simulink model "Vertiport_performance"  (R2022b)
settings: Solver=VariableStepAuto  StartTime=0.0  StopTime=1080  RelTol=1e-3
model workspace (MAT data in the model file):
  ChargingRate = 5
  MinTurnAround = 5
  ReqBatteryLevel = 70
  SeparationMinima = 3
  UAMDemand = 183
undefined symbols (not defined in the file or in its folder): entity, m, n, recordWaitTimes
settings Model: Creator=user  LastModifiedBy=user
settings SolverCC: AlgebraicLoopSolver=TrustRegion
settings DataIOCC: SaveOutput=off  SaveTime=off
settings DebuggingCC: UnconnectedInputMsg=warning  UnconnectedOutputMsg=warning  UnconnectedLineMsg=warning  SFMachineParentedDataDiag=warning  ArithmeticOperatorsInVariantConditions=warning
settings ModelReferenceCC: EnableRefExpFcnMdlSchedulingChecks=on
settings SFSimCC: SimUseLocalCustomCode=off  CustomCodeUndefinedFunction=UseInterfaceOnly
settings RTWCC: RTWUseLocalCustomCode=off
settings CodeAppCC: StateflowObjectComments=on

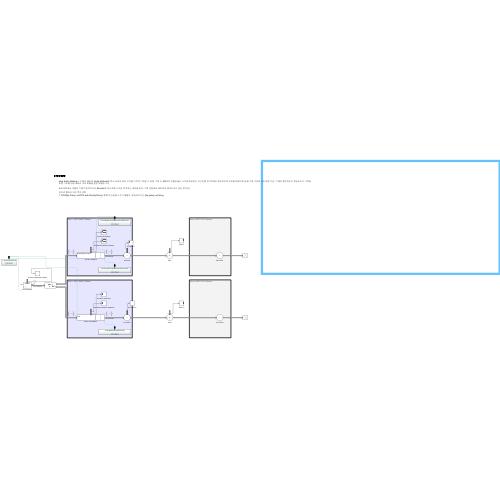
[thumbnail: Simulink's stored preview of the top-level diagram]
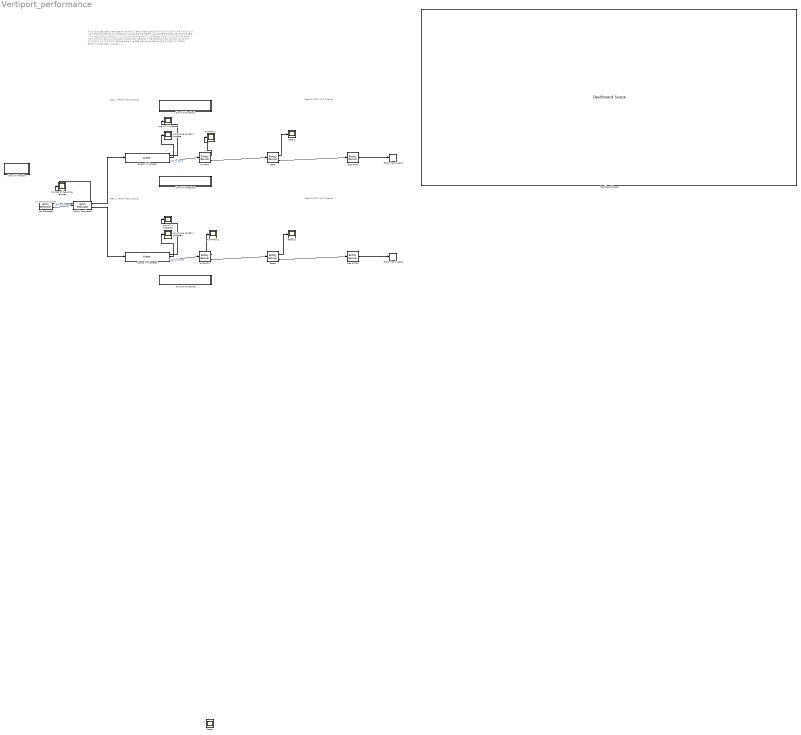
== system Vertiport_performance ==
  note: 27.7920676732485
  note: Step 3: FATO [·/D/1 Queue]
  note: Step 1: FATO [M/D/1 Queue]
  note: ※ 향후 방향
      |
      | Idea: Entity Attribute = 기체의 배터리, Entity Attribute에 따라 서버의 점유 시간을 다르게 가져갈 수 있음, 가령 1~100까지 만들어놓고 그거에 해당하는 시간만큼 게이트에서 점유하도록 규칙을 배정하면 실제 기체 거리에 따라 배정 가능. 기체의 충전속도는 동일하다고 가정 & 비행 거리에 따른 배터리 소모 비율을 알면 모델링 가능
      |
      | 버티포트에서 어떻게 기체가 움직이는지 Simulink로 모사해주고 이걸 분석하는 내용을 담자. 기체 관점에서 버티포트 에어사이드 성능 분석(?)
      |
      | 앞으로 뽑아야 하는 분석 방향
      | 1. FIFO(No Policy) vs FIFO with Priority(Policy): 통행 우선권을 가진 기체들의 평균대기시간 (No policy vs Policy),
  note: Step 1: FATO [M/D/1 Queue]
  note: Step 3: FATO [·/D/1 Queue]
  " Avg Queue Length in Airspace" : Scope
  " Avg Queue Length in Airspace1" : Scope
  Arr FATO : EntityServer  InputPortMessageModes=m  OutputPortMessageModes=n,m  Capacity=1  ServiceTimeSource=MATLAB action  ServiceTimeValue=1.5  ServiceTimeAction=dt = SeparationMinima;  Utilization=on
      settings: OutputPortMap=o5,o9
  Arr FATO U : Scope
  Arr FATO U1 : Scope
  Arr FATO1 : EntityServer  InputPortMessageModes=m  OutputPortMessageModes=n,m  Capacity=1  ServiceTimeSource=MATLAB action  ServiceTimeValue=1.5  ServiceTimeAction=dt = SeparationMinima;  Utilization=on
      settings: OutputPortMap=o5,o9
  Avg WT in Airspace : Scope
  Avg WT in Airspace1 : Scope
  Dashboard Scope : DashboardScope
  Dep FATO : EntityServer  InputPortMessageModes=m  OutputPortMessageModes=m  Capacity=1  ServiceTimeSource=MATLAB action  ServiceTimeAction=dt = SeparationMinima;
  Dep FATO1 : EntityServer  InputPortMessageModes=m  OutputPortMessageModes=m  Capacity=1  ServiceTimeSource=MATLAB action  ServiceTimeAction=dt = SeparationMinima;
  Entity Replicator : EntityReplicator  InputPortMessageModes=m  OutputPortMessageModes=m,m
  Entity Terminator1 : EntityTerminator  InputPortMessageModes=m
  Entity Terminator2 : EntityTerminator  InputPortMessageModes=m
  Gate : EntityServer  InputPortMessageModes=m  OutputPortMessageModes=n,m  ServiceTimeSource=MATLAB action  ServiceTimeValue=20  ServiceTimeAction=|  ServiceCompleteAction=|  Utilization=on
      ServiceTimeAction=|
      | if ReqBatteryLevel <= entity.Battery ...
      |         + MinTurnAround*ChargingRate
      |     dt = MinTurnAround;
      | else
      |     dt = (ReqBatteryLevel - entity.Battery)/ChargingRate
      | end
      ServiceCompleteAction=|
      | if entity.Battery >= ReqBatteryLevel - MinTurnAround*ChargingRate
      |     entity.Battery = min(100, entity.Battery + MinTurnAround*ChargingRate);
      | else
      |     entity.Battery = ReqBatteryLevel;
      | end
      settings: OutputPortMap=o5,o9
  Gate U : Scope
  Gate U1 : Scope
  Gate1 : EntityServer  InputPortMessageModes=m  OutputPortMessageModes=n,m  ServiceTimeSource=MATLAB action  ServiceTimeValue=20  ServiceTimeAction=|  ServiceCompleteAction=|  Utilization=on
      ServiceTimeAction=|
      | if ReqBatteryLevel <= entity.Battery ...
      |         + MinTurnAround*ChargingRate
      |     dt = MinTurnAround;
      | else
      |     dt = (ReqBatteryLevel - entity.Battery)/ChargingRate
      | end
      ServiceCompleteAction=|
      | if entity.Battery >= ReqBatteryLevel - MinTurnAround*ChargingRate
      |     entity.Battery = min(100, entity.Battery + MinTurnAround*ChargingRate);
      | else
      |     entity.Battery = ReqBatteryLevel;
      | end
      settings: OutputPortMap=o5,o9
  Number of departing vehicles : Scope
  Queue in Airspace : Queue  InputPortMessageModes=m  OutputPortMessageModes=n,n,m  Capacity=50  QueueType=Priority  PrioritySource=entitySys.priority  EntryAction=entity.StartTime = getCurrentTime();  ExitAction=|  AverageWait=on  AverageQueueLength=on
      | if entity.Class == 1
      |     recordHighPriorityWaitTimes(...
      |     entity.StartTime);
      | else
      |     recordLowPriorityWaitTimes(...
      |     entity.StartTime)
      | end % if entity.Class = 1
      settings: OutputPortMap=o2,o3,o5
  Queue in Airspace1 : Queue  InputPortMessageModes=m  OutputPortMessageModes=n,n,m  Capacity=50  PrioritySource=entitySys.priority  EntryAction=entity.StartTime = getCurrentTime();  ExitAction=recordWaitTimes(entity.StartTime)  AverageWait=on  AverageQueueLength=on
      settings: OutputPortMap=o2,o3,o5
  Simulink Function : Subsystem  TreatAsAtomicUnit=on
  Simulink Function1 : Subsystem  TreatAsAtomicUnit=on
  Simulink Function2 : Subsystem  TreatAsAtomicUnit=on
  Simulink Function5 : Subsystem  TreatAsAtomicUnit=on
  Veh Generator : EntityGenerator  OutputPortMessageModes=n,m  TimeSource=MATLAB action  IntergenerationTimeAction=|  GenerateEntityAtSimulationStart=off  GenerateAction=|  AttributeName=Battery|Class|StartTime  AttributeInitialValue=1|2|1  NumberEntitiesDeparted=on  EntityType=Structured  EntityTypeName=Vehicle
      IntergenerationTimeAction=|
      | persistent rngInit;
      | if isempty(rngInit)
      |     seed = 12345;
      |     rng(seed);
      |     rngInit = true;
      | end
      | 
      | B = [0.0361866444691084, 0.105565575286718, 0.157539076951535, 0.0409961154273030, 0.0182898631150573,0.0195847206807251, 0.0247930540140585, 0.0321113115057344, 0.0338628375878653, 0.0467131428042915, 0.0718472530521643, 0.0986172770995191, 0.121190575286718, 0.0568118756936737, 0.0477363115057344, 0.0432447743248243, 0.0326373473917869, 0.0122722438031817]';
      | Length = size(B,1);
      | UAMDemandHr = UAMDemand.*B(:,1);
      | Time = 60
      | Now = getCurrentTime();
      | aa = mod(Now, (Time*Length));
      | k = 1 + floor(aa./Time);
      | ArrivalRate = UAMDemandHr(k,1);
      | 
      | % Pattern: Exponential distribution
      | mu = 60/ArrivalRate; % mu = avg(interarrival time)
      | dt = - mu * log(1 - rand());
      GenerateAction=|
      | entity.Battery = randi(80);
      | % 배터리 1~80 까지 임의 생성
      | % 배터리 10미만이면 통행 우선권 부여
      | % 우버에서 minimum reserve 30%로 제
      | 
      | if entity.Battery <= 10
      |     entity.Class = 1;
      | else
      |     entity.Class = 2;
      | end % if entity.Battery < 10
      | 
      | entitySys.priority = entity.Class;
      settings: OutputPortMap=o0,o3
  Scope : Scope
  wires:
  Gate/2 -> Dep FATO/1
  Queue in Airspace/1 -> Avg WT in Airspace/1
  Arr FATO/2 -> Gate/1
  Queue in Airspace/3 -> Arr FATO/1  "Veh to FATO"
  Queue in Airspace/2 -> " Avg Queue Length in Airspace"/1
  Gate/1 -> Gate U/1
  Dep FATO/1 -> Entity Terminator1/1
  Veh Generator/2 -> Entity Replicator/1  "Veh to Airspace"
  Queue in Airspace1/2 -> " Avg Queue Length in Airspace1"/1
  Queue in Airspace1/3 -> Arr FATO1/1  "Veh to FATO1"
  Dep FATO1/1 -> Entity Terminator2/1
  Gate1/2 -> Dep FATO1/1
  Gate1/1 -> Gate U1/1
  Queue in Airspace1/1 -> Avg WT in Airspace1/1
  Entity Replicator/1 -> Queue in Airspace/1
  Entity Replicator/2 -> Queue in Airspace1/1
  Arr FATO/1 -> Arr FATO U/1
  Arr FATO1/1 -> Arr FATO U1/1
  Veh Generator/1 -> Number of departing vehicles/1
  Arr FATO1/2 -> Gate1/1

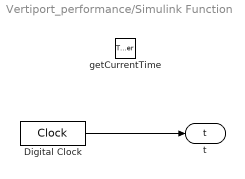
== system Vertiport_performance/Simulink Function ==
  getCurrentTime : TriggerPort  TriggerType=function-call  IsSimulinkFunction=on  FunctionName=getCurrentTime  VariantControl=Variant
  Digital Clock : DigitalClock  SampleTime=-1
  t : ArgOut  DisableCoverage=on  ArgumentName=t
  wires:
  Digital Clock/1 -> t/1

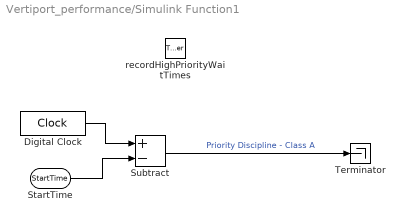
== system Vertiport_performance/Simulink Function1 ==
  recordHighPriorityWaitTimes : TriggerPort  TriggerType=function-call  IsSimulinkFunction=on  FunctionName=recordHighPriorityWaitTimes  VariantControl=Variant
  Digital Clock : DigitalClock  SampleTime=-1
  Subtract : Sum  Inputs=+-
  Terminator : Terminator
  StartTime : ArgIn  DisableCoverage=on  ArgumentName=StartTime
  wires:
  StartTime/1 -> Subtract/2
  Digital Clock/1 -> Subtract/1
  Subtract/1 -> Terminator/1  "Priority Discipline - Class A"

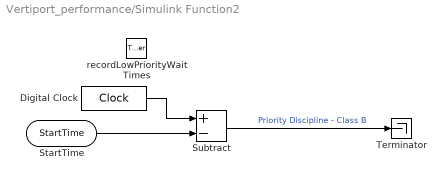
== system Vertiport_performance/Simulink Function2 ==
  recordLowPriorityWaitTimes : TriggerPort  TriggerType=function-call  IsSimulinkFunction=on  FunctionName=recordLowPriorityWaitTimes  VariantControl=Variant
  Digital Clock : DigitalClock  SampleTime=-1
  Subtract : Sum  Inputs=+-
  Terminator : Terminator
  StartTime : ArgIn  DisableCoverage=on  ArgumentName=StartTime
  wires:
  StartTime/1 -> Subtract/2
  Digital Clock/1 -> Subtract/1
  Subtract/1 -> Terminator/1  "Priority Discipline - Class B"

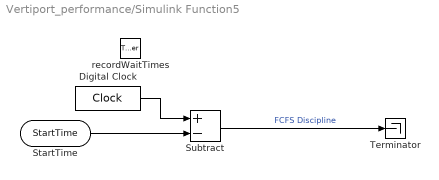
== system Vertiport_performance/Simulink Function5 ==
  recordWaitTimes : TriggerPort  TriggerType=function-call  IsSimulinkFunction=on  FunctionName=recordWaitTimes  VariantControl=Variant
  Digital Clock : DigitalClock  SampleTime=-1
  Subtract : Sum  Inputs=+-
  Terminator : Terminator
  StartTime : ArgIn  DisableCoverage=on  ArgumentName=StartTime
  wires:
  StartTime/1 -> Subtract/2
  Digital Clock/1 -> Subtract/1
  Subtract/1 -> Terminator/1  "FCFS Discipline"
